simulink subsystem "Porportional_Follower"  (R2022b)
settings: Solver=VariableStepAuto  StartTime=0.0  StopTime=10.0  RelTol=1e-3
settings Model: Creator=hollis  LastModifiedBy=hollis

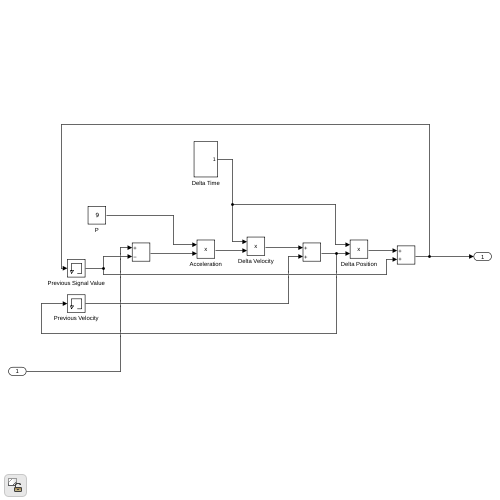
[thumbnail: Simulink's stored preview of the top-level diagram]
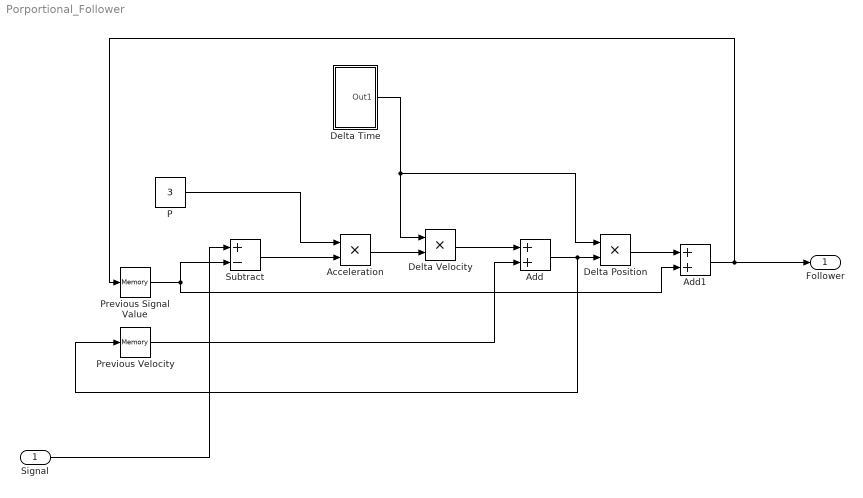
== system Porportional_Follower ==
  Signal : Inport
  Acceleration : Product
  Add : Sum
  Add1 : Sum
  Delta Position : Product
  Delta Time : Subsystem
  Delta Velocity : Product
  P : Constant  Value=3
  Previous Signal Value : Memory
  Previous Velocity : Memory
  Subtract : Sum  Inputs=+-
  Follower : Outport
  wires:
  P/1 -> Acceleration/1
  Signal/1 -> Subtract/1
  Previous Signal Value/1 -> Add1/2, Subtract/2
  Subtract/1 -> Acceleration/2
  Acceleration/1 -> Delta Velocity/2
  Delta Time/1(Out1) -> Delta Velocity/1, Delta Position/1
  Previous Velocity/1 -> Add/2
  Delta Velocity/1 -> Add/1
  Add/1 -> Delta Position/2, Previous Velocity/1
  Delta Position/1 -> Add1/1
  Add1/1 -> Previous Signal Value/1, Follower/1

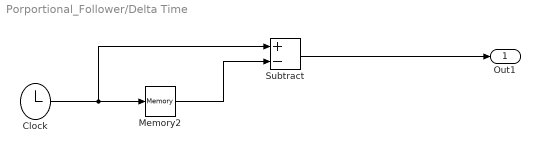
== system Porportional_Follower/Delta Time ==
  Clock : Clock
  Memory2 : Memory
  Subtract : Sum  Inputs=+-
  Out1 : Outport
  wires:
  Subtract/1 -> Out1/1
  Clock/1 -> Memory2/1, Subtract/1
  Memory2/1 -> Subtract/2
